simulink model "Model_Calibration"  (R2021a)
settings: Solver=ode4  StartTime=0.0  StopTime=tend  FixedStep=dt  RelTol=1e-3
values from neighbouring files (symbols this model uses):
  A_cplant = plantFRAME_SS.a    [S2_Plant_Ref_Part.m]
  B_cplant = plantFRAME_SS.b    [S2_Plant_Ref_Part.m]
  C_cplant = plantFRAME_SS.c    [S2_Plant_Ref_Part.m]
  correction_gain1 = 1.053    [S1_Input_Data.m]
  correction_gain2 = 1.055    [S1_Input_Data.m]
  D_cplant = plantFRAME_SS.d    [S2_Plant_Ref_Part.m]
  dt = 1/fs    [S1_Input_Data.m]
  EQ_intensity = intensities(j)    [Offline_calibration.m]
  sat_limit = 3.8    [S1_Input_Data.m]
  Seed_snr = rng(seed)    [S1_Input_Data.m]
  v2d_const1 = 0.0092    [S1_Input_Data.m]
  v2d_const2 = -0.0059    [S1_Input_Data.m]
  v2d_gain1 = 7.4921    [S1_Input_Data.m]
  v2d_gain2 = 7.3907    [S1_Input_Data.m]
undefined symbols (not defined in the file or in its folder): a0, a1, a2, a3, a4, a5, a6, a7, AgN, alpha1, alpha2, CNrt, dv1, dv2, EQ_sw, FN, KNbar_inv, lN, MNrt, RNbar
libraries: simulink x2
settings Model: Creator=icu327  LastModifiedBy=maryf
settings SolverCC: AlgebraicLoopSolver=TrustRegion
settings DataIOCC: SaveFormat=Array  ReturnWorkspaceOutputs=off
settings DebuggingCC: ArithmeticOperatorsInVariantConditions=warning
settings SFSimCC: CustomCodeUndefinedFunction=UseInterfaceOnly
settings RTWCC: Description=Simulink Desktop Real-Time  SystemTargetFile=sldrt.tlc  TemplateMakefile=sldrt.tmf  RTWCompilerOptimization=on
settings CodeAppCC: MaxIdLength=95  StateflowObjectComments=on
settings SimulinkDesktopRealTimeCC: TargetPreCompLibLocation=C:\Program Files\MATLAB\R2021a\toolbox\sldrt\lib\win64

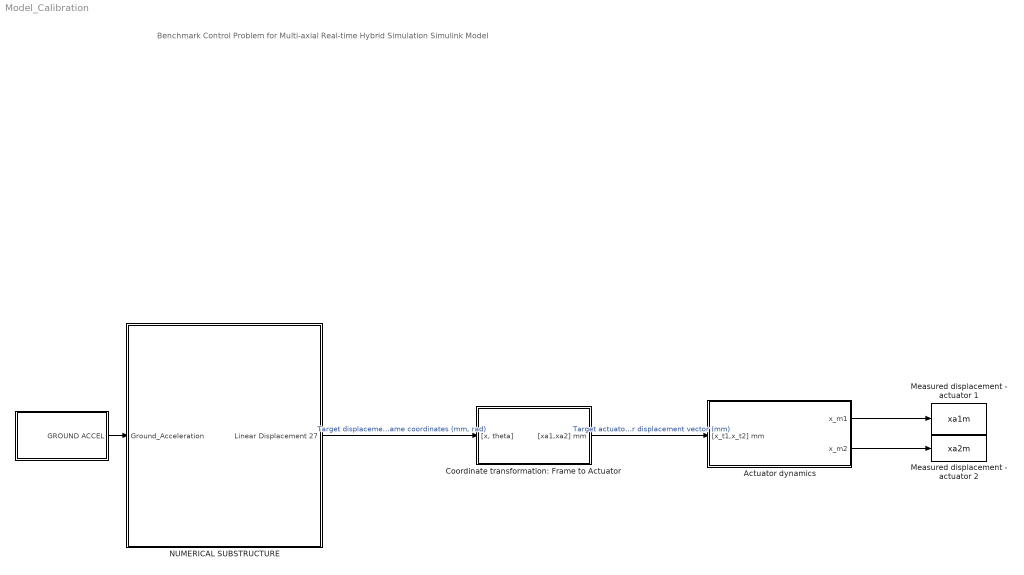
== system Model_Calibration ==
  note: Benchmark Control Problem for Multi-axial Real-time Hybrid Simulation
      | Simulink Model
  " " : Subsystem
  " NUMERICAL SUBSTRUCTURE" : Subsystem
      mask Display: image('$imagefile'); % Use "Edit Image" on toolstrip to change.
  Actuator dynamics : Subsystem
  Coordinate transformation: Frame to Actuator : Subsystem
  Measured displacement - actuator 1 : ToWorkspace  VariableName=xa1m  SampleTime=dt
  Measured displacement - actuator 2 : ToWorkspace  VariableName=xa2m  SampleTime=dt
  wires:
  " "/1(GROUND ACCEL) -> " NUMERICAL SUBSTRUCTURE"/1(Ground_Acceleration)
  Coordinate transformation: Frame to Actuator/1("[xa1,xa2] mm") -> Actuator dynamics/1("[x_t1,x_t2] mm")  "Target actuator displacement vector (mm)"
  " NUMERICAL SUBSTRUCTURE"/1(Linear Displacement 27) -> Coordinate transformation: Frame to Actuator/1("[x, theta]")  "Target displacement vector Frame coordinates (mm, rad)"
  Actuator dynamics/1(x_m1) -> Measured displacement - actuator 1/1
  Actuator dynamics/2(x_m2) -> Measured displacement - actuator 2/1

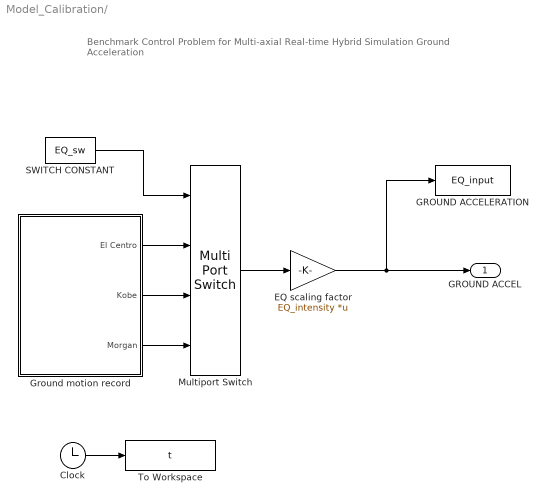
== system Model_Calibration/  ==
  note: Benchmark Control Problem for
      | Multi-axial Real-time Hybrid Simulation
      | Ground Acceleration
  Clock : Clock
  EQ scaling factor : Gain  Gain=EQ_intensity  Multiplication=Matrix(K*u)
  GROUND ACCELERATION : ToWorkspace  VariableName=EQ_input  SampleTime=-1
      settings: Save2DSignal=2-D array (concatenate along first dimension)
  Ground motion record : Subsystem
  Multiport Switch : MultiPortSwitch
  SWITCH CONSTANT : Constant  Value=EQ_sw
  To Workspace : ToWorkspace  VariableName=t  SampleTime=dt
  GROUND ACCEL : Outport  VectorParamsAs1DForOutWhenUnconnected=off
  wires:
  Multiport Switch/1 -> EQ scaling factor/1
  EQ scaling factor/1 -> GROUND ACCELERATION/1, GROUND ACCEL/1
  Ground motion record/1(El Centro) -> Multiport Switch/2
  Ground motion record/2(Kobe) -> Multiport Switch/3
  Ground motion record/3(Morgan) -> Multiport Switch/4
  SWITCH CONSTANT/1 -> Multiport Switch/1
  Clock/1 -> To Workspace/1

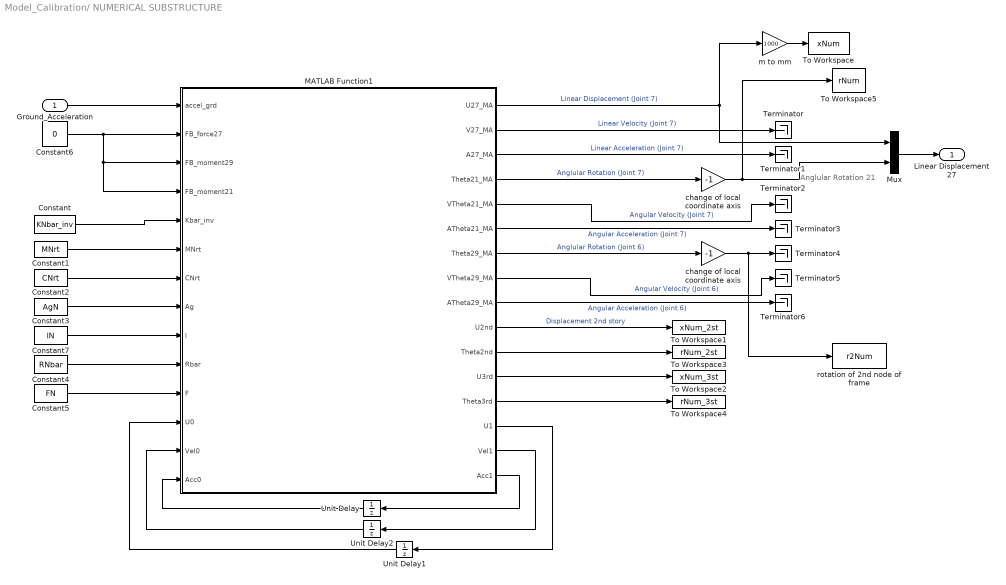
== system Model_Calibration/ NUMERICAL SUBSTRUCTURE ==
  note: Anglular Rotation 21
  Ground_Acceleration : Inport
  Constant : Constant  Value=KNbar_inv  VectorParams1D=off
  Constant1 : Constant  Value=MNrt  VectorParams1D=off
  Constant2 : Constant  Value=CNrt  VectorParams1D=off
  Constant3 : Constant  Value=AgN  VectorParams1D=off
  Constant4 : Constant  Value=RNbar  VectorParams1D=off
  Constant5 : Constant  Value=FN  VectorParams1D=off
  Constant6 : Constant  Value=0
  Constant7 : Constant  Value=lN  VectorParams1D=off
  MATLAB Function1 : MATLAB Function  TreatAsAtomicUnit=on
  Mux : Mux  Inputs=2
  Terminator{,1..6} (7 alike) : Terminator
  To Workspace : ToWorkspace  VariableName=xNum  SampleTime=dt
  To Workspace1 : ToWorkspace  VariableName=xNum_2st  SampleTime=dt
  To Workspace2 : ToWorkspace  VariableName=xNum_3st  SampleTime=dt
  To Workspace3 : ToWorkspace  VariableName=rNum_2st  SampleTime=dt
  To Workspace4 : ToWorkspace  VariableName=rNum_3st  SampleTime=dt
  To Workspace5 : ToWorkspace  VariableName=rNum  SampleTime=dt
  Unit Delay : UnitDelay  SampleTime=-1  HasFrameUpgradeWarning=on
  Unit Delay1 : UnitDelay  SampleTime=-1  HasFrameUpgradeWarning=on
  Unit Delay2 : UnitDelay  SampleTime=-1  HasFrameUpgradeWarning=on
  change of local coordinate axis : Gain  Gain=-1
  "change of local coordinate axis  " : Gain  Gain=-1
  "m to mm " : Gain  Gain=1000
  rotation of 2nd node of frame : ToWorkspace  VariableName=r2Num  SampleTime=dt
      settings: Tag=rst
  Linear Displacement 27 : Outport  VectorParamsAs1DForOutWhenUnconnected=off
  wires:
  Ground_Acceleration/1 -> MATLAB Function1/1(accel_grd)
  MATLAB Function1/1(U27_MA) -> Mux/1, "m to mm "/1  "Linear Displacement (Joint 7)"
  MATLAB Function1/4(Theta21_MA) -> change of local coordinate axis/1  "Anglular Rotation (Joint 7)"
  Constant/1 -> MATLAB Function1/5(Kbar_inv)
  Constant1/1 -> MATLAB Function1/6(MNrt)
  Constant2/1 -> MATLAB Function1/7(CNrt)
  Constant3/1 -> MATLAB Function1/8(Ag)
  Constant7/1 -> MATLAB Function1/9(l)
  Constant4/1 -> MATLAB Function1/10(Rbar)
  Unit Delay1/1 -> MATLAB Function1/12(U0)
  Unit Delay2/1 -> MATLAB Function1/13(Vel0)
  Unit Delay/1 -> MATLAB Function1/14(Acc0)
  MATLAB Function1/15(Vel1) -> Unit Delay2/1
  MATLAB Function1/16(Acc1) -> Unit Delay/1
  MATLAB Function1/14(U1) -> Unit Delay1/1
  Constant5/1 -> MATLAB Function1/11(F)
  MATLAB Function1/2(V27_MA) -> Terminator/1  "Linear Velocity (Joint 7)"
  MATLAB Function1/3(A27_MA) -> Terminator1/1  "Linear Acceleration (Joint 7)"
  MATLAB Function1/5(VTheta21_MA) -> Terminator2/1  "Angular Velocity (Joint 7)"
  MATLAB Function1/6(ATheta21_MA) -> Terminator3/1  "Angular Acceleration (Joint 7)"
  MATLAB Function1/9(ATheta29_MA) -> Terminator6/1  "Angular Acceleration (Joint 6)"
  MATLAB Function1/8(VTheta29_MA) -> Terminator5/1  "Angular Velocity (Joint 6)"
  MATLAB Function1/7(Theta29_MA) -> "change of local coordinate axis  "/1  "Anglular Rotation (Joint 6)"
  Constant6/1 -> MATLAB Function1/4(FB_moment21), MATLAB Function1/3(FB_moment29), MATLAB Function1/2(FB_force27)
  MATLAB Function1/10(U2nd) -> To Workspace1/1  "Displacement 2nd story"
  MATLAB Function1/11(Theta2nd) -> To Workspace3/1
  MATLAB Function1/12(U3rd) -> To Workspace2/1
  MATLAB Function1/13(Theta3rd) -> To Workspace4/1
  "m to mm "/1 -> To Workspace/1
  change of local coordinate axis/1 -> Mux/2, To Workspace5/1
  "change of local coordinate axis  "/1 -> Terminator4/1, rotation of 2nd node of frame/1
  Mux/1 -> Linear Displacement 27/1

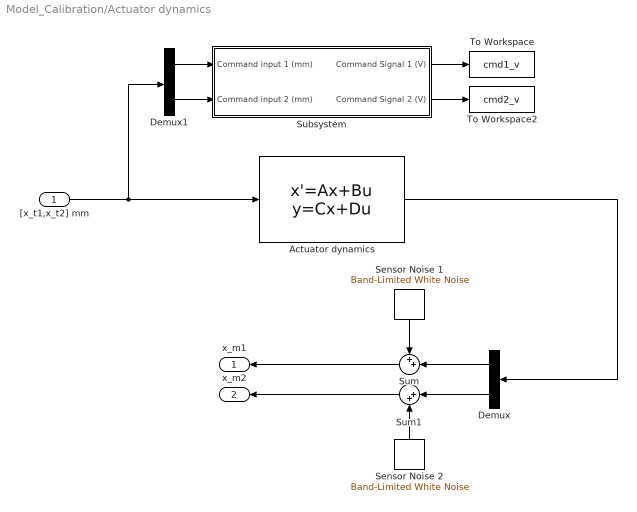
== system Model_Calibration/Actuator dynamics ==
  "[x_t1,x_t2] mm" : Inport
  Actuator dynamics : StateSpace  A=A_cplant  B=B_cplant  C=C_cplant  D=D_cplant  InitialCondition=0
  Demux : Demux  Outputs=2
  Demux1 : Demux  Outputs=2
  Sensor Noise 1 : simulink/Sources/Band-Limited White Noise  Cov=rms_noise_DT  Ts=dt  seed=double(Seed_snr.Seed)
  Sensor Noise 2 : simulink/Sources/Band-Limited White Noise  Cov=rms_noise_DT  Ts=dt  seed=double(Seed_snr.Seed)
  Subsystem : Subsystem
  Sum : Sum  Inputs=++|
  Sum1 : Sum  Inputs=|++
  To Workspace : ToWorkspace  VariableName=cmd1_v  SampleTime=dt
  To Workspace2 : ToWorkspace  VariableName=cmd2_v  SampleTime=dt
  x_m1 : Outport
  x_m2 : Outport  Port=2
  wires:
  Actuator dynamics/1 -> Demux/1
  "[x_t1,x_t2] mm"/1 -> Demux1/1, Actuator dynamics/1
  Demux/2 -> Sum1/1
  Demux/1 -> Sum/2
  Subsystem/1(Command Signal 1 (V)) -> To Workspace/1
  Demux1/2 -> Subsystem/2(Command input 2 (mm))
  Demux1/1 -> Subsystem/1(Command input 1 (mm))
  Subsystem/2(Command Signal 2 (V)) -> To Workspace2/1
  Sensor Noise 1/1 -> Sum/1
  Sensor Noise 2/1 -> Sum1/2
  Sum/1 -> x_m1/1
  Sum1/1 -> x_m2/1

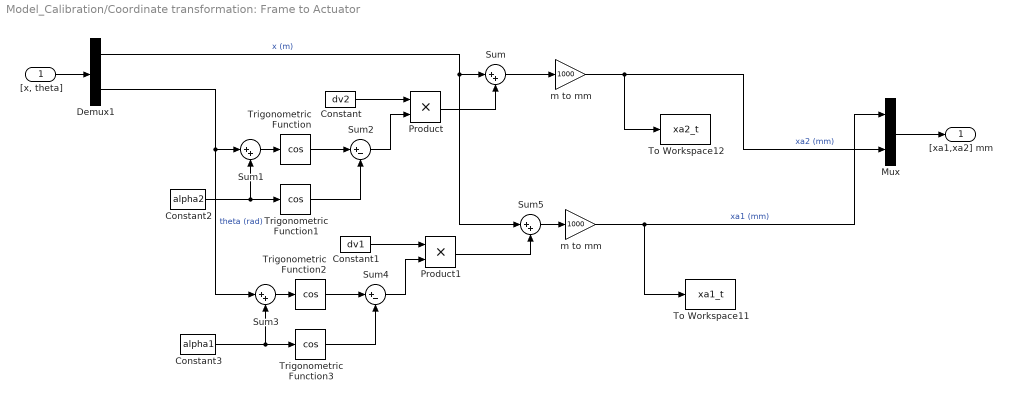
== system Model_Calibration/Coordinate transformation: Frame to Actuator ==
  "[x, theta]" : Inport
  Constant : Constant  Value=dv2
  Constant1 : Constant  Value=dv1
  Constant2 : Constant  Value=alpha2
  Constant3 : Constant  Value=alpha1
  Demux1 : Demux  Outputs=2
  Mux : Mux  Inputs=2
  Product : Product
  Product1 : Product
  Sum{,1,3,5} (4 alike) : Sum  Inputs=|++
  Sum2 : Sum  Inputs=|+-
  Sum4 : Sum  Inputs=|+-
  To Workspace11 : ToWorkspace  VariableName=xa1_t  SampleTime=dt
  To Workspace12 : ToWorkspace  VariableName=xa2_t  SampleTime=dt
  Trigonometric Function{,1..3} (4 alike) : Trigonometry  Operator=cos
  m to mm : Gain  Gain=1000
  "m to mm " : Gain  Gain=1000
  "[xa1,xa2] mm" : Outport  VectorParamsAs1DForOutWhenUnconnected=off
  wires:
  Constant/1 -> Product/1
  Constant2/1 -> Sum1/2, Trigonometric Function1/1
  Sum1/1 -> Trigonometric Function/1
  Trigonometric Function/1 -> Sum2/1
  Trigonometric Function1/1 -> Sum2/2
  Sum2/1 -> Product/2
  Product/1 -> Sum/2
  Sum/1 -> m to mm/1
  Sum4/1 -> Product1/2
  Trigonometric Function3/1 -> Sum4/2
  Trigonometric Function2/1 -> Sum4/1
  Sum3/1 -> Trigonometric Function2/1
  Constant3/1 -> Sum3/2, Trigonometric Function3/1
  Constant1/1 -> Product1/1
  Product1/1 -> Sum5/2
  Sum5/1 -> "m to mm "/1
  "m to mm "/1 -> To Workspace11/1, Mux/1  "xa1 (mm)"
  m to mm/1 -> To Workspace12/1, Mux/2  "xa2 (mm)"
  Demux1/1 -> Sum/1, Sum5/1  "x (m)"
  "[x, theta]"/1 -> Demux1/1
  Demux1/2 -> Sum3/1, Sum1/1  "theta (rad)"
  Mux/1 -> "[xa1,xa2] mm"/1

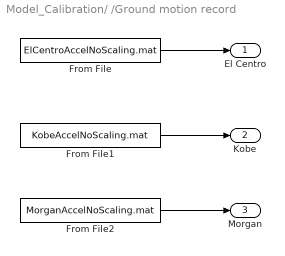
== system Model_Calibration/ /Ground motion record ==
  From File : FromFile  FileName=ElCentroAccelNoScaling.mat  SampleTime=dt
  From File1 : FromFile  FileName=KobeAccelNoScaling.mat  SampleTime=dt
  From File2 : FromFile  FileName=MorganAccelNoScaling.mat  SampleTime=dt
  El Centro : Outport
  Kobe : Outport  Port=2
  Morgan : Outport  Port=3
  wires:
  From File/1 -> El Centro/1
  From File2/1 -> Morgan/1
  From File1/1 -> Kobe/1

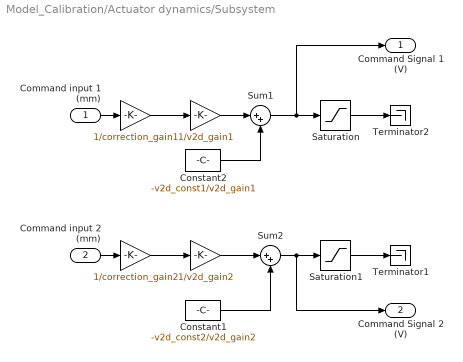
== system Model_Calibration/Actuator dynamics/Subsystem ==
  Command input 1 (mm) : Inport
  Command input 2 (mm) : Inport  Port=2
  " " : Gain  Gain=1/v2d_gain2
  "  " : Gain  Gain=1/v2d_gain1
  "   " : Gain  Gain=1/correction_gain1
  "    " : Gain  Gain=1/correction_gain2
  Constant1 : Constant  Value=-v2d_const2/v2d_gain2
  Constant2 : Constant  Value=-v2d_const1/v2d_gain1
  Saturation : Saturate  UpperLimit=sat_limit  LowerLimit=-sat_limit
  Saturation1 : Saturate  UpperLimit=sat_limit  LowerLimit=-sat_limit
  Sum1 : Sum  Inputs=|++
  Sum2 : Sum  Inputs=|++
  Terminator1 : Terminator
  Terminator2 : Terminator
  Command Signal 1 (V) : Outport  VectorParamsAs1DForOutWhenUnconnected=off
  Command Signal 2 (V) : Outport  Port=2  VectorParamsAs1DForOutWhenUnconnected=off
  wires:
  "   "/1 -> "  "/1
  Command input 1 (mm)/1 -> "   "/1
  Constant1/1 -> Sum2/2
  " "/1 -> Sum2/1
  Constant2/1 -> Sum1/2
  "  "/1 -> Sum1/1
  Sum1/1 -> Command Signal 1 (V)/1, Saturation/1
  "    "/1 -> " "/1
  Sum2/1 -> Command Signal 2 (V)/1, Saturation1/1
  Command input 2 (mm)/1 -> "    "/1
  Saturation/1 -> Terminator2/1
  Saturation1/1 -> Terminator1/1

== matlab function Model_Calibration/ NUMERICAL SUBSTRUCTURE/MATLAB Function1 ==
  data: U27_MA output; V27_MA output; A27_MA output; Theta21_MA output; VTheta21_MA output; ATheta21_MA output; Theta29_MA output; VTheta29_MA output; ATheta29_MA output; U2nd output; Theta2nd output; U3rd output; Theta3rd output; U1 output; Vel1 output; Acc1 output; accel_grd input; FB_force27 input; FB_moment29 input; FB_moment21 input; Kbar_inv input; MNrt input; CNrt input; Ag input; l input; Rbar input; F input; U0 input; Vel0 input; Acc0 input; a0 parameter; a1 parameter; a2 parameter; a3 parameter; a4 parameter; a5 parameter; a6 parameter; a7 parameter
function [U27_MA,V27_MA,A27_MA,Theta21_MA,VTheta21_MA,ATheta21_MA,Theta29_MA,VTheta29_MA,ATheta29_MA,U2nd,Theta2nd,U3rd,Theta3rd,U1,Vel1,Acc1]=...
    fcn(accel_grd,FB_force27,FB_moment29,FB_moment21,Kbar_inv, MNrt, CNrt,Ag,l,Rbar,F,...
    U0,Vel0,Acc0, a0, a1, a2, a3, a4, a5, a6, a7)
             
             
    % ============================
	% *  Update next iteration   *
	% ============================
    ndof = length(Kbar_inv);
    U1   = zeros(ndof,1);
    Vel1 = zeros(ndof,1);
    Acc1 = zeros(ndof,1);
    
    U27_MA = 0;
    V27_MA = 0;
    A27_MA = 0;

    Theta21_MA = 0;
    VTheta21_MA = 0;
    ATheta21_MA = 0;
% 
%     U6_MA = 0;
%     V6_MA = 0;
%     A6_MA = 0;
    U2nd = 0 ;              %Displacement 2nd story, node 12, DOF 26
    Theta2nd = 0;          %Rotation 2nd story, node 12, DOF 22
    U3rd = 0;              %Displacement 3rd story, node 16, DOF 13
    Theta3rd = 0;           %Rotation 3rd story, node 16, DOF 3


    Theta29_MA = 0;
    VTheta29_MA = 0;
    ATheta29_MA = 0;

    % ============================
	% *  Feedback Force / Moment *
	% ============================
    F(27) = FB_force27;
    F(21) = FB_moment21;
    F(29) = FB_moment29;

    % ==========================
	% *     Update Matrices    *
	% ==========================
    Ag(:)  = accel_grd * l;
    
   	% ==========================
	% * 	  Form Rbar  	   *
	% ==========================
	Rbar = ( (MNrt * ((a0*U0)+(a2*Vel0)+(a3*Acc0))) + ...
		     (CNrt * ((a1*U0)+(a4*Vel0)+(a5*Acc0))) - F - (MNrt * Ag) );
    
    % ==========================
	% * Solve for Displacement *
	% ==========================
	U1 = Kbar_inv * Rbar;
    
	% ============================
	% * Compute Velocity & Accel *
	% ============================
	Acc1=a0*(U1-U0)-a2*Vel0-a3*Acc0;
	Vel1=Vel0+a7*Acc1+a6*Acc0; 

	% ============================
	% *    Output u1 and theta   *
	% ============================
    U27_MA    = U1(27);
    V27_MA    = Vel1(27);
    A27_MA    = Acc1(27);    

%     U6_MA    = U1(27);
%     V6_MA    = Vel1(27);
%     A6_MA    = Acc1(27);

    Theta21_MA = U1(21);
    VTheta21_MA = Vel1(21);
    ATheta21_MA = Acc1(21);

    Theta29_MA = U1(29);
    VTheta29_MA = Vel1(29);
    ATheta29_MA = Acc1(29);
    
    % ADDED by Johnny
    U2nd = U1(26);              %Displacement 2nd story, node 12, DOF 26
    Theta2nd = U1(22);          %Rotation 2nd story, node 12, DOF 22
    U3rd = U1(13);              %Displacement 3rd story, node 16, DOF 13
    Theta3rd = U1(3);           %Rotation 3rd story, node 16, DOF 3

end
